simulink model "simulation"  (R2022b)
settings: Solver=ode4  StartTime=0.0  StopTime=10.0  FixedStep=0.01  RelTol=1e-3
undefined symbols (not defined in the file or in its folder): DiscIntNeverNeededParam, r, v
settings Model: Creator=lulav  LastModifiedBy=lulav

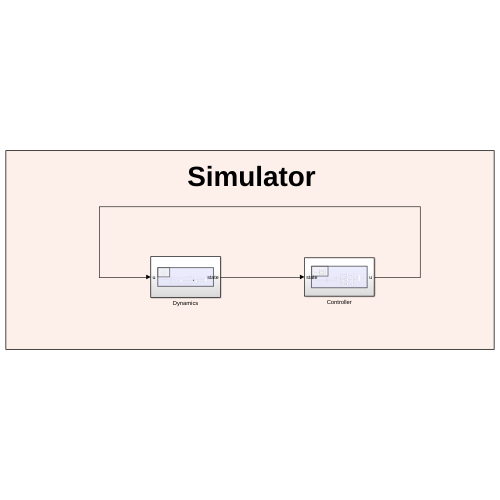
[thumbnail: Simulink's stored preview of the top-level diagram]
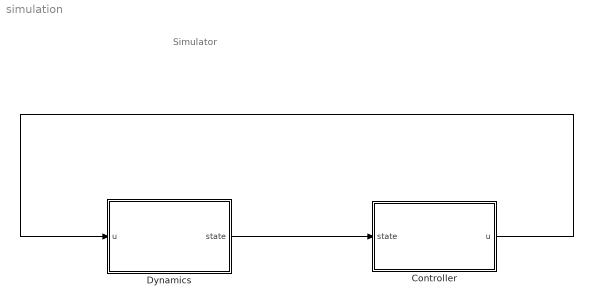
== system simulation ==
  note: Simulator
  Controller : Subsystem
  Dynamics : Subsystem
  wires:
  Dynamics/1(state) -> Controller/1(state)
  Controller/1(u) -> Dynamics/1(u)

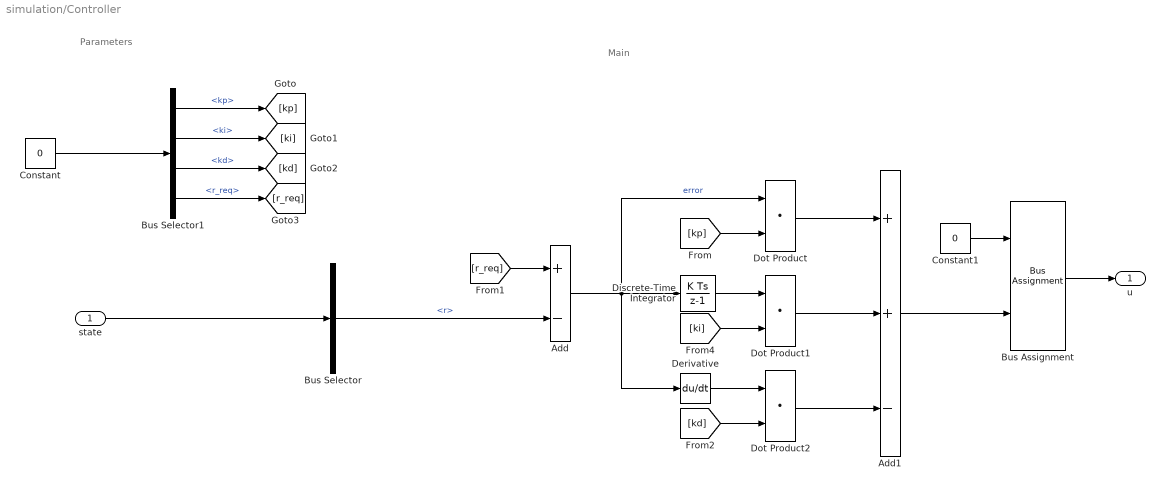
== system simulation/Controller ==
  note: Main
  note: Parameters
  state : Inport  OutDataTypeStr=Bus: Dynamics
  Add : Sum  Inputs=+-
  Add1 : Sum  Inputs=++-
  Bus Assignment : BusAssignment  AssignedSignals=u
  Bus Selector : BusSelector  OutputSignals=r
  Bus Selector1 : BusSelector  OutputSignals=kp,ki,kd,r_req
  Constant : Constant  Value=0  OutDataTypeStr=Bus: Params
  Constant1 : Constant  Value=0  OutDataTypeStr=Bus: Controller
  Derivative : Derivative
  Discrete-Time Integrator : DiscreteIntegrator  SampleTime=-1  ICPrevOutput=DiscIntNeverNeededParam  ICPrevScaledInput=DiscIntNeverNeededParam
  Dot Product : DotProduct  OutDataTypeStr=Inherit: Inherit via internal rule
  Dot Product1 : DotProduct  OutDataTypeStr=Inherit: Inherit via internal rule
  Dot Product2 : DotProduct  OutDataTypeStr=Inherit: Inherit via internal rule
  u : Outport  OutDataTypeStr=Bus: Controller
  wires:
  Bus Selector1/3 -> [kd]  "<kd>"
  Constant/1 -> Bus Selector1/1
  Bus Selector1/4 -> [r_req]  "<r_req>"
  state/1 -> Bus Selector/1
  Bus Selector1/2 -> [ki]  "<ki>"
  Bus Selector1/1 -> [kp]  "<kp>"
  Bus Selector/1 -> Add/2  "<r>"
  [r_req] -> Add/1
  Add/1 -> Discrete-Time Integrator/1, Dot Product/1, Derivative/1  "error"
  Discrete-Time Integrator/1 -> Dot Product1/1
  Derivative/1 -> Dot Product2/1
  [kp] -> Dot Product/2
  [ki] -> Dot Product1/2
  [kd] -> Dot Product2/2
  Dot Product/1 -> Add1/1
  Dot Product1/1 -> Add1/2
  Dot Product2/1 -> Add1/3
  Add1/1 -> Bus Assignment/2
  Bus Assignment/1 -> u/1
  Constant1/1 -> Bus Assignment/1

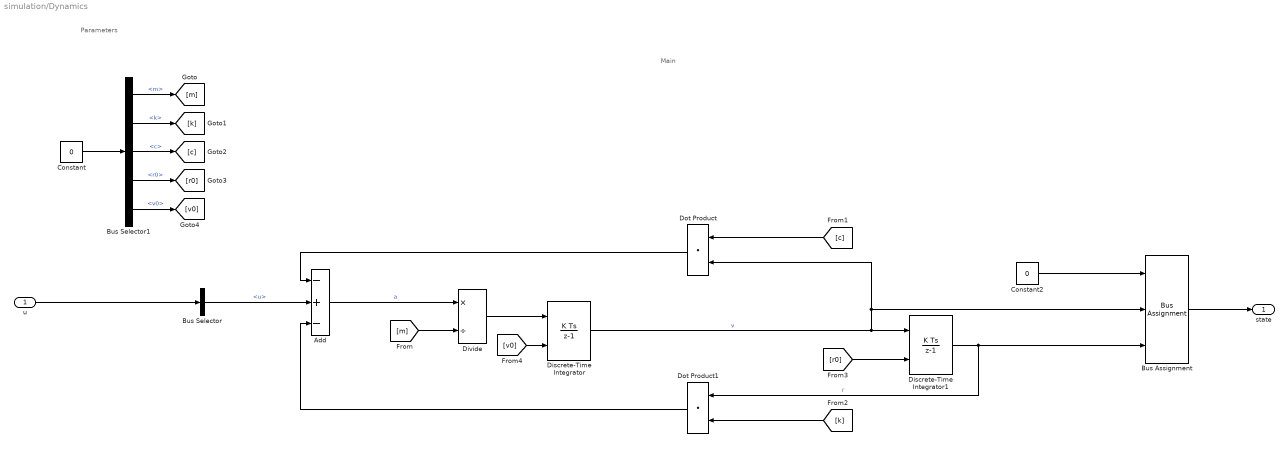
== system simulation/Dynamics ==
  note: Main
  note: Parameters
  u : Inport  OutDataTypeStr=Bus: Controller
  Add : Sum  Inputs=-+-
  Bus Assignment : BusAssignment  AssignedSignals=v,r
  Bus Selector : BusSelector  OutputSignals=u
  Bus Selector1 : BusSelector  OutputSignals=m,k,c,r0,v0
  Constant : Constant  Value=0  OutDataTypeStr=Bus: Params
  Constant2 : Constant  Value=0  OutDataTypeStr=Bus: Dynamics
  Discrete-Time Integrator : DiscreteIntegrator  InitialConditionSource=external  SampleTime=-1  ICPrevOutput=DiscIntNeverNeededParam  ICPrevScaledInput=DiscIntNeverNeededParam
  Discrete-Time Integrator1 : DiscreteIntegrator  InitialConditionSource=external  SampleTime=-1  ICPrevOutput=DiscIntNeverNeededParam  ICPrevScaledInput=DiscIntNeverNeededParam
  Divide : Product  Inputs=*/
  Dot Product : DotProduct  OutDataTypeStr=Inherit: Inherit via internal rule
  Dot Product1 : DotProduct  OutDataTypeStr=Inherit: Inherit via internal rule
  state : Outport  OutDataTypeStr=Bus: Dynamics
  wires:
  Constant/1 -> Bus Selector1/1
  Bus Selector1/5 -> [v0]  "<v0>"
  Dot Product1/1 -> Add/3
  Divide/1 -> Discrete-Time Integrator/1
  Bus Selector1/4 -> [r0]  "<r0>"
  Bus Assignment/1 -> state/1
  [r0] -> Discrete-Time Integrator1/2
  Discrete-Time Integrator/1 -> Discrete-Time Integrator1/1, Dot Product/2, Bus Assignment/2  "v"
  Add/1 -> Divide/1  "a"
  Constant2/1 -> Bus Assignment/1
  [c] -> Dot Product/1
  Discrete-Time Integrator1/1 -> Dot Product1/1, Bus Assignment/3  "r"
  Bus Selector1/3 -> [c]  "<c>"
  [v0] -> Discrete-Time Integrator/2
  [k] -> Dot Product1/2
  Dot Product/1 -> Add/1
  Bus Selector1/1 -> [m]  "<m>"
  Bus Selector1/2 -> [k]  "<k>"
  u/1 -> Bus Selector/1
  [m] -> Divide/2
  Bus Selector/1 -> Add/2  "<u>"
